simulink model "testupdate"  (R2014b)
settings: Solver=ode1  StartTime=0.0  StopTime=10.0  FixedStep=.1  RelTol=1e-3
undefined symbols (not defined in the file or in its folder): stateA
settings Model: Creator=emiller  LastModifiedBy=emiller

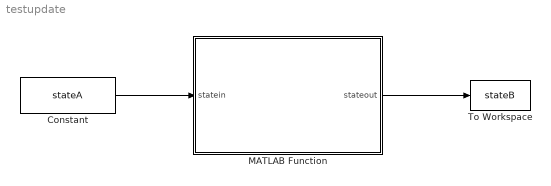
== system testupdate ==
  Constant : Constant  Value=stateA  OutDataTypeStr=Bus: stateAbus
  MATLAB Function : MATLAB Function  TreatAsAtomicUnit=on
  To Workspace : ToWorkspace  VariableName=stateB  SaveFormat=Timeseries  SampleTime=-1
  wires:
  Constant/1 -> MATLAB Function/1(statein)
  MATLAB Function/1(stateout) -> To Workspace/1

== matlab function testupdate/MATLAB Function ==
  data: statein input Bus: stateAbus; stateout output Bus: stateAbus
function stateout = UpdateState(statein)
%#codegen

stateout=statein;
fluid=stateout.fluid;

%Define Pressure and Specific Enthalpy
p=stateout.pressure;
h=stateout.enthalpy./stateout.mass;

%Interpolation
stateout.temperature=interp2(fluid.P,fluid.H,fluid.TPH,p,h);
stateout.density=interp2(fluid.P,fluid.H,fluid.DPH,p,h);
stateout.quality=interp2(fluid.P,fluid.H,fluid.QPH,p,h);
